simulink model "gimbal_test_2017_11_24"  (R2017a)
settings: Solver=ode14x  StartTime=0.0  StopTime=20  FixedStep=0.001  RelTol=1e-3  EnableMultiTasking=on
values from neighbouring files (symbols this model uses):
  m = MAG(:,3:5)    [acc_calibration_t1.m]
  s = tf('s')    [adaptive_control.m]    (also in constraints.m = 1e-19)
undefined symbols (not defined in the file or in its folder): sigbuilder_block, X, Y, Z
libraries: sm_lib x46, nesl_utility x35, simulink x7
(part 2 of 2)

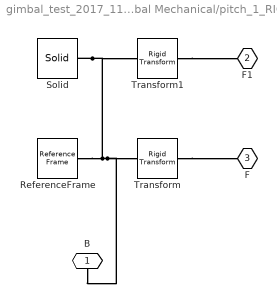
== system gimbal_test_2017_11_24/Gimbal Mechanical/pitch_1_RIGID ==
  ReferenceFrame : sm_lib/Frames and Transforms/Reference Frame
  Solid : sm_lib/Body Elements/Solid  InertiaType=Custom  Mass=0.14119942872953756  MassUnits=kg  CenterOfMass=[-40.309869373451356 137.87074734557396 -65.780666800490948]  CenterOfMassUnits=mm  MomentsOfInertia=[409.04449997922234 176.99414095993797 350.83879275246994]  MomentsOfInertiaUnits=kg*mm^2  ProductsOfInertia=[-106.85964081398967 1.9282234630967596 4.2232275028540895]  ProductsOfInertiaUnits=kg*mm^2  DensityBased=on  Density=1000  DensityUnits=kg/(m^3)  DoExposeReferenceFrame=on  SerializedFrames=<Frames/>  GraphicType=FromGeometry  MarkerShape=Sphere  MarkerSize=10  GraphicVisPropType=SimpleVisualProperties  GraphicDiffuseColor=[0.89803921568627454 0.91764705882352937 0.92941176470588238]  GraphicSpecularColor=[0.5 0.5 0.5 1.0]  GraphicAmbientColor=[0.15 0.15 0.15 1.0]  GraphicEmissiveColor=[0.0 0.0 0.0 1.0]  GraphicShininess=75  GraphicOpacity=1  GeometryShape=FromFile  RectangleSize=[1 1]  RectangleSizeUnits=m  BrickDimensions=[1 1 1]  BrickDimensionUnits=m  CylinderRadius=1  CylinderRadiusUnits=m  CylinderLength=1  CylinderLengthUnits=m  SphereRadius=1  SphereRadiusUnits=m  EllipsoidRadii=[1 1 1]  EllipsoidRadiiUnits=m  ExtrusionCrossSection=[1 1; -1 1; -1 -1; 1 -1]  ExtrusionCrossSectionUnits=m  ExtrusionLength=1  ExtrusionLengthUnits=m  PolygonNumSides=3  PolygonOuterRadius=1  PolygonOuterRadiusUnits=m  ExtGeomFileType=STEP  ExtGeomFileName=pitch_默认_sldprt.STEP  ExtGeomFileUnits=m  RevolutionCrossSection=[1 1; 1 -1; 2 -1; 2 1]  RevolutionCrossSectionUnits=m  RevolutionExtent=Full  RevolutionAngle=180  RevolutionAngleUnits=deg
  Transform : sm_lib/Frames and Transforms/Rigid Transform  TranslationMethod=Cartesian  TranslationStandardOffset=0  TranslationLengthUnit=mm  TranslationStandardAxis=+Z  TranslationCartesianOffset=[-70.90915967289996 155.67572530099997 -91.396390597699934]  TranslationROffset=0  TranslationROffsetUnits=m  TranslationZOffset=0  TranslationZOffsetUnits=m  TranslationThetaOffset=0  TranslationThetaOffsetUnits=deg  RotationMethod=ArbitraryAxis  RotationAngleUnits=rad  RotationStandardAxis=+Z  RotationAngle=0  RotationArbitraryAxis=[0 0 0]  FollAlignAxisA=+X  BaseAlignAxisA=+Y  FollAlignAxisB=+Y  BaseAlignAxisB=+Z  RotationSequenceAxes=FollowerAxes  RotationSequence=XYX  RotationSequenceAngles=[0 0 0]  RotationSequenceAnglesUnits=deg  RotationMatrix=[1 0 0; 0 1 0; 0 0 1]
  Transform1 : sm_lib/Frames and Transforms/Rigid Transform  TranslationMethod=Cartesian  TranslationStandardOffset=0  TranslationLengthUnit=mm  TranslationStandardAxis=+Z  TranslationCartesianOffset=[-38.909159672900159 1166.6150256647427 -32.030390597696254]  TranslationROffset=0  TranslationROffsetUnits=m  TranslationZOffset=0  TranslationZOffsetUnits=m  TranslationThetaOffset=0  TranslationThetaOffsetUnits=deg  RotationMethod=ArbitraryAxis  RotationAngleUnits=rad  RotationStandardAxis=+Z  RotationAngle=2.0943951023931957  RotationArbitraryAxis=[0.57735026918962595 -0.57735026918962595 0.5773502691896254]  FollAlignAxisA=+X  BaseAlignAxisA=+Y  FollAlignAxisB=+Y  BaseAlignAxisB=+Z  RotationSequenceAxes=FollowerAxes  RotationSequence=XYX  RotationSequenceAngles=[0 0 0]  RotationSequenceAnglesUnits=deg  RotationMatrix=[1 0 0; 0 1 0; 0 0 1]
  B : PMIOPort  Port=1  Side=Left
  F1 : PMIOPort  Port=2  Side=Left
  F : PMIOPort  Port=3  Side=Left
  connections:
  Solid/RConn1 -- B/RConn1 -- Transform/LConn1 -- Transform1/LConn1 -- ReferenceFrame/RConn1
  Transform/RConn1 -- F/RConn1
  Transform1/RConn1 -- F1/RConn1

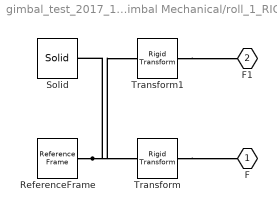
== system gimbal_test_2017_11_24/Gimbal Mechanical/roll_1_RIGID ==
  ReferenceFrame : sm_lib/Frames and Transforms/Reference Frame
  Solid : sm_lib/Body Elements/Solid  InertiaType=Custom  Mass=0.31793228993235328  MassUnits=kg  CenterOfMass=[-40.197559372662035 151.39080125157062 -75.482343271011416]  CenterOfMassUnits=mm  MomentsOfInertia=[1698.578771208184 766.33943967936329 1161.8382457192142]  MomentsOfInertiaUnits=kg*mm^2  ProductsOfInertia=[-589.52899840909799 -20.442997774547614 -29.224073948839539]  ProductsOfInertiaUnits=kg*mm^2  DensityBased=on  Density=1000  DensityUnits=kg/(m^3)  DoExposeReferenceFrame=on  SerializedFrames=<Frames/>  GraphicType=FromGeometry  MarkerShape=Sphere  MarkerSize=10  GraphicVisPropType=SimpleVisualProperties  GraphicDiffuseColor=[0.89803921568627454 0.91764705882352937 0.92941176470588238]  GraphicSpecularColor=[0.5 0.5 0.5 1.0]  GraphicAmbientColor=[0.15 0.15 0.15 1.0]  GraphicEmissiveColor=[0.0 0.0 0.0 1.0]  GraphicShininess=75  GraphicOpacity=1  GeometryShape=FromFile  RectangleSize=[1 1]  RectangleSizeUnits=m  BrickDimensions=[1 1 1]  BrickDimensionUnits=m  CylinderRadius=1  CylinderRadiusUnits=m  CylinderLength=1  CylinderLengthUnits=m  SphereRadius=1  SphereRadiusUnits=m  EllipsoidRadii=[1 1 1]  EllipsoidRadiiUnits=m  ExtrusionCrossSection=[1 1; -1 1; -1 -1; 1 -1]  ExtrusionCrossSectionUnits=m  ExtrusionLength=1  ExtrusionLengthUnits=m  PolygonNumSides=3  PolygonOuterRadius=1  PolygonOuterRadiusUnits=m  ExtGeomFileType=STEP  ExtGeomFileName=roll_默认_sldprt.STEP  ExtGeomFileUnits=m  RevolutionCrossSection=[1 1; 1 -1; 2 -1; 2 1]  RevolutionCrossSectionUnits=m  RevolutionExtent=Full  RevolutionAngle=180  RevolutionAngleUnits=deg
  Transform : sm_lib/Frames and Transforms/Rigid Transform  TranslationMethod=Cartesian  TranslationStandardOffset=0  TranslationLengthUnit=mm  TranslationStandardAxis=+Z  TranslationCartesianOffset=[-38.909159672899136 47.175725301000313 513.35498149905948]  TranslationROffset=0  TranslationROffsetUnits=m  TranslationZOffset=0  TranslationZOffsetUnits=m  TranslationThetaOffset=0  TranslationThetaOffsetUnits=deg  RotationMethod=ArbitraryAxis  RotationAngleUnits=rad  RotationStandardAxis=+Z  RotationAngle=3.1415926535897931  RotationArbitraryAxis=[-1 1.5338031114433573e-32 -2.7175667253946204e-16]  FollAlignAxisA=+X  BaseAlignAxisA=+Y  FollAlignAxisB=+Y  BaseAlignAxisB=+Z  RotationSequenceAxes=FollowerAxes  RotationSequence=XYX  RotationSequenceAngles=[0 0 0]  RotationSequenceAnglesUnits=deg  RotationMatrix=[1 0 0; 0 1 0; 0 0 1]
  Transform1 : sm_lib/Frames and Transforms/Rigid Transform  TranslationMethod=Cartesian  TranslationStandardOffset=0  TranslationLengthUnit=mm  TranslationStandardAxis=+Z  TranslationCartesianOffset=[-38.909159672900039 1167.1810510685002 -32.030390597700006]  TranslationROffset=0  TranslationROffsetUnits=m  TranslationZOffset=0  TranslationZOffsetUnits=m  TranslationThetaOffset=0  TranslationThetaOffsetUnits=deg  RotationMethod=ArbitraryAxis  RotationAngleUnits=rad  RotationStandardAxis=+Z  RotationAngle=2.0943951023931953  RotationArbitraryAxis=[0.57735026918962584 -0.57735026918962584 0.57735026918962584]  FollAlignAxisA=+X  BaseAlignAxisA=+Y  FollAlignAxisB=+Y  BaseAlignAxisB=+Z  RotationSequenceAxes=FollowerAxes  RotationSequence=XYX  RotationSequenceAngles=[0 0 0]  RotationSequenceAnglesUnits=deg  RotationMatrix=[1 0 0; 0 1 0; 0 0 1]
  F : PMIOPort  Port=1  Side=Left
  F1 : PMIOPort  Port=2  Side=Right
  connections:
  Solid/RConn1 -- ReferenceFrame/RConn1 -- Transform/LConn1 -- Transform1/LConn1
  Transform/RConn1 -- F/RConn1
  Transform1/RConn1 -- F1/RConn1

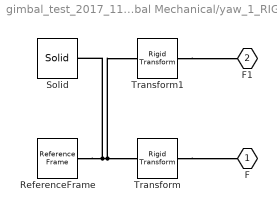
== system gimbal_test_2017_11_24/Gimbal Mechanical/yaw_1_RIGID ==
  ReferenceFrame : sm_lib/Frames and Transforms/Reference Frame
  Solid : sm_lib/Body Elements/Solid  InertiaType=Custom  Mass=0.4220224652422469  MassUnits=kg  CenterOfMass=[-39.730395407906954 147.5203430562342 -125.35459490281445]  CenterOfMassUnits=mm  MomentsOfInertia=[6109.2729904538583 920.66918616811347 5510.6384164735264]  MomentsOfInertiaUnits=kg*mm^2  ProductsOfInertia=[-1282.9600428246124 21.67357327564007 52.078346871971853]  ProductsOfInertiaUnits=kg*mm^2  DensityBased=on  Density=1000  DensityUnits=kg/(m^3)  DoExposeReferenceFrame=on  SerializedFrames=<Frames/>  GraphicType=FromGeometry  MarkerShape=Sphere  MarkerSize=10  GraphicVisPropType=SimpleVisualProperties  GraphicDiffuseColor=[0.89803921568627454 0.91764705882352937 0.92941176470588238]  GraphicSpecularColor=[0.5 0.5 0.5 1.0]  GraphicAmbientColor=[0.15 0.15 0.15 1.0]  GraphicEmissiveColor=[0.0 0.0 0.0 1.0]  GraphicShininess=75  GraphicOpacity=1  GeometryShape=FromFile  RectangleSize=[1 1]  RectangleSizeUnits=m  BrickDimensions=[1 1 1]  BrickDimensionUnits=m  CylinderRadius=1  CylinderRadiusUnits=m  CylinderLength=1  CylinderLengthUnits=m  SphereRadius=1  SphereRadiusUnits=m  EllipsoidRadii=[1 1 1]  EllipsoidRadiiUnits=m  ExtrusionCrossSection=[1 1; -1 1; -1 -1; 1 -1]  ExtrusionCrossSectionUnits=m  ExtrusionLength=1  ExtrusionLengthUnits=m  PolygonNumSides=3  PolygonOuterRadius=1  PolygonOuterRadiusUnits=m  ExtGeomFileType=STEP  ExtGeomFileName=yaw_默认_sldprt.STEP  ExtGeomFileUnits=m  RevolutionCrossSection=[1 1; 1 -1; 2 -1; 2 1]  RevolutionCrossSectionUnits=m  RevolutionExtent=Full  RevolutionAngle=180  RevolutionAngleUnits=deg
  Transform : sm_lib/Frames and Transforms/Rigid Transform  TranslationMethod=Cartesian  TranslationStandardOffset=0  TranslationLengthUnit=mm  TranslationStandardAxis=+Z  TranslationCartesianOffset=[-38.909159672899804 334.03951901900109 -32.030390597700091]  TranslationROffset=0  TranslationROffsetUnits=m  TranslationZOffset=0  TranslationZOffsetUnits=m  TranslationThetaOffset=0  TranslationThetaOffsetUnits=deg  RotationMethod=ArbitraryAxis  RotationAngleUnits=rad  RotationStandardAxis=+Z  RotationAngle=2.0943951023931962  RotationArbitraryAxis=[0.57735026918962595 -0.57735026918962562 0.57735026918962573]  FollAlignAxisA=+X  BaseAlignAxisA=+Y  FollAlignAxisB=+Y  BaseAlignAxisB=+Z  RotationSequenceAxes=FollowerAxes  RotationSequence=XYX  RotationSequenceAngles=[0 0 0]  RotationSequenceAnglesUnits=deg  RotationMatrix=[1 0 0; 0 1 0; 0 0 1]
  Transform1 : sm_lib/Frames and Transforms/Rigid Transform  TranslationMethod=Cartesian  TranslationStandardOffset=0  TranslationLengthUnit=mm  TranslationStandardAxis=+Z  TranslationCartesianOffset=[-38.909159672900067 32.039519019000039 520.28895609530014]  TranslationROffset=0  TranslationROffsetUnits=m  TranslationZOffset=0  TranslationZOffsetUnits=m  TranslationThetaOffset=0  TranslationThetaOffsetUnits=deg  RotationMethod=ArbitraryAxis  RotationAngleUnits=rad  RotationStandardAxis=+Z  RotationAngle=3.1415926535897931  RotationArbitraryAxis=[1 0 5.377642775528102e-17]  FollAlignAxisA=+X  BaseAlignAxisA=+Y  FollAlignAxisB=+Y  BaseAlignAxisB=+Z  RotationSequenceAxes=FollowerAxes  RotationSequence=XYX  RotationSequenceAngles=[0 0 0]  RotationSequenceAnglesUnits=deg  RotationMatrix=[1 0 0; 0 1 0; 0 0 1]
  F : PMIOPort  Port=1  Side=Left
  F1 : PMIOPort  Port=2  Side=Right
  connections:
  Solid/RConn1 -- ReferenceFrame/RConn1 -- Transform/LConn1 -- Transform1/LConn1
  Transform/RConn1 -- F/RConn1
  Transform1/RConn1 -- F1/RConn1

== system gimbal_test_2017_11_24/Test Bed/groud_1_RIGID ==
  ReferenceFrame : sm_lib/Frames and Transforms/Reference Frame
  Solid : sm_lib/Body Elements/Solid  InertiaType=Custom  Mass=0.744656095436107  MassUnits=kg  CenterOfMass=[0 14.834199182049298 0]  CenterOfMassUnits=mm  MomentsOfInertia=[248.52962199765179 383.88524366097863 245.75166872905808]  MomentsOfInertiaUnits=kg*mm^2  ProductsOfInertia=[0 0 0]  ProductsOfInertiaUnits=kg*mm^2  DensityBased=on  Density=1000  DensityUnits=kg/(m^3)  DoExposeReferenceFrame=on  SerializedFrames=<Frames/>  GraphicType=FromGeometry  MarkerShape=Sphere  MarkerSize=10  GraphicVisPropType=SimpleVisualProperties  GraphicDiffuseColor=[0.89411764705882346 0.9137254901960784 0.92941176470588238]  GraphicSpecularColor=[0.5 0.5 0.5 1.0]  GraphicAmbientColor=[0.15 0.15 0.15 1.0]  GraphicEmissiveColor=[0.0 0.0 0.0 1.0]  GraphicShininess=75  GraphicOpacity=1  GeometryShape=FromFile  RectangleSize=[1 1]  RectangleSizeUnits=m  BrickDimensions=[1 1 1]  BrickDimensionUnits=m  CylinderRadius=1  CylinderRadiusUnits=m  CylinderLength=1  CylinderLengthUnits=m  SphereRadius=1  SphereRadiusUnits=m  EllipsoidRadii=[1 1 1]  EllipsoidRadiiUnits=m  ExtrusionCrossSection=[1 1; -1 1; -1 -1; 1 -1]  ExtrusionCrossSectionUnits=m  ExtrusionLength=1  ExtrusionLengthUnits=m  PolygonNumSides=3  PolygonOuterRadius=1  PolygonOuterRadiusUnits=m  ExtGeomFileType=STEP  ExtGeomFileName=groud_默认_sldprt.STEP  ExtGeomFileUnits=m  RevolutionCrossSection=[1 1; 1 -1; 2 -1; 2 1]  RevolutionCrossSectionUnits=m  RevolutionExtent=Full  RevolutionAngle=180  RevolutionAngleUnits=deg
  Transform : sm_lib/Frames and Transforms/Rigid Transform  TranslationMethod=Cartesian  TranslationStandardOffset=0  TranslationLengthUnit=mm  TranslationStandardAxis=+Z  TranslationCartesianOffset=[0 30 0]  TranslationROffset=0  TranslationROffsetUnits=m  TranslationZOffset=0  TranslationZOffsetUnits=m  TranslationThetaOffset=0  TranslationThetaOffsetUnits=deg  RotationMethod=ArbitraryAxis  RotationAngleUnits=rad  RotationStandardAxis=+Z  RotationAngle=2.0943951023931953  RotationArbitraryAxis=[0.57735026918962584 -0.57735026918962584 0.57735026918962584]  FollAlignAxisA=+X  BaseAlignAxisA=+Y  FollAlignAxisB=+Y  BaseAlignAxisB=+Z  RotationSequenceAxes=FollowerAxes  RotationSequence=XYX  RotationSequenceAngles=[0 0 0]  RotationSequenceAnglesUnits=deg  RotationMatrix=[1 0 0; 0 1 0; 0 0 1]
  F1 : PMIOPort  Port=1  Side=Left
  F : PMIOPort  Port=2  Side=Right
  connections:
  Solid/RConn1 -- ReferenceFrame/RConn1 -- Transform/LConn1 -- F1/RConn1
  Transform/RConn1 -- F/RConn1

== system gimbal_test_2017_11_24/Test Bed/test_pitch_1_RIGID ==
  ReferenceFrame : sm_lib/Frames and Transforms/Reference Frame
  Solid : sm_lib/Body Elements/Solid  InertiaType=Custom  Mass=3.2542558482698221  MassUnits=kg  CenterOfMass=[0 15.000000000000004 0.00013445046945364221]  CenterOfMassUnits=mm  MomentsOfInertia=[197323.97689125084 354318.98035563418 157585.85549691919]  MomentsOfInertiaUnits=kg*mm^2  ProductsOfInertia=[0 0 0.0039657370023979469]  ProductsOfInertiaUnits=kg*mm^2  DensityBased=on  Density=1000  DensityUnits=kg/(m^3)  DoExposeReferenceFrame=on  SerializedFrames=<Frames/>  GraphicType=FromGeometry  MarkerShape=Sphere  MarkerSize=10  GraphicVisPropType=SimpleVisualProperties  GraphicDiffuseColor=[1 1 1]  GraphicSpecularColor=[0.5 0.5 0.5 1.0]  GraphicAmbientColor=[0.15 0.15 0.15 1.0]  GraphicEmissiveColor=[0.0 0.0 0.0 1.0]  GraphicShininess=75  GraphicOpacity=1  GeometryShape=FromFile  RectangleSize=[1 1]  RectangleSizeUnits=m  BrickDimensions=[1 1 1]  BrickDimensionUnits=m  CylinderRadius=1  CylinderRadiusUnits=m  CylinderLength=1  CylinderLengthUnits=m  SphereRadius=1  SphereRadiusUnits=m  EllipsoidRadii=[1 1 1]  EllipsoidRadiiUnits=m  ExtrusionCrossSection=[1 1; -1 1; -1 -1; 1 -1]  ExtrusionCrossSectionUnits=m  ExtrusionLength=1  ExtrusionLengthUnits=m  PolygonNumSides=3  PolygonOuterRadius=1  PolygonOuterRadiusUnits=m  ExtGeomFileType=STEP  ExtGeomFileName=test_pitch_默认_sldprt.STEP  ExtGeomFileUnits=m  RevolutionCrossSection=[1 1; 1 -1; 2 -1; 2 1]  RevolutionCrossSectionUnits=m  RevolutionExtent=Full  RevolutionAngle=180  RevolutionAngleUnits=deg
  Transform : sm_lib/Frames and Transforms/Rigid Transform  TranslationMethod=Cartesian  TranslationStandardOffset=0  TranslationLengthUnit=mm  TranslationStandardAxis=+Z  TranslationCartesianOffset=[0 15.000000000000568 -587]  TranslationROffset=0  TranslationROffsetUnits=m  TranslationZOffset=0  TranslationZOffsetUnits=m  TranslationThetaOffset=0  TranslationThetaOffsetUnits=deg  RotationMethod=ArbitraryAxis  RotationAngleUnits=rad  RotationStandardAxis=+Z  RotationAngle=8.3312973296909746e-16  RotationArbitraryAxis=[0.86265645032380789 -0.50579032089861853 -1.8175695005807099e-16]  FollAlignAxisA=+X  BaseAlignAxisA=+Y  FollAlignAxisB=+Y  BaseAlignAxisB=+Z  RotationSequenceAxes=FollowerAxes  RotationSequence=XYX  RotationSequenceAngles=[0 0 0]  RotationSequenceAnglesUnits=deg  RotationMatrix=[1 0 0; 0 1 0; 0 0 1]
  Transform1 : sm_lib/Frames and Transforms/Rigid Transform  TranslationMethod=Cartesian  TranslationStandardOffset=0  TranslationLengthUnit=mm  TranslationStandardAxis=+Z  TranslationCartesianOffset=[0 30 0]  TranslationROffset=0  TranslationROffsetUnits=m  TranslationZOffset=0  TranslationZOffsetUnits=m  TranslationThetaOffset=0  TranslationThetaOffsetUnits=deg  RotationMethod=ArbitraryAxis  RotationAngleUnits=rad  RotationStandardAxis=+Z  RotationAngle=2.0943951023931953  RotationArbitraryAxis=[0.57735026918962584 -0.57735026918962584 0.57735026918962584]  FollAlignAxisA=+X  BaseAlignAxisA=+Y  FollAlignAxisB=+Y  BaseAlignAxisB=+Z  RotationSequenceAxes=FollowerAxes  RotationSequence=XYX  RotationSequenceAngles=[0 0 0]  RotationSequenceAnglesUnits=deg  RotationMatrix=[1 0 0; 0 1 0; 0 0 1]
  F : PMIOPort  Port=1  Side=Left
  F1 : PMIOPort  Port=2  Side=Right
  connections:
  Solid/RConn1 -- ReferenceFrame/RConn1 -- Transform/LConn1 -- Transform1/LConn1
  Transform/RConn1 -- F/RConn1
  Transform1/RConn1 -- F1/RConn1

== system gimbal_test_2017_11_24/Test Bed/test_roll_1_RIGID ==
  ReferenceFrame : sm_lib/Frames and Transforms/Reference Frame
  Solid : sm_lib/Body Elements/Solid  InertiaType=Custom  Mass=0.20450614916336574  MassUnits=kg  CenterOfMass=[-1.0328761560106987e-05 10.226639389930648 -309.12731029151979]  CenterOfMassUnits=mm  MomentsOfInertia=[71.504553359544801 477.13713336271184 448.94842380562415]  MomentsOfInertiaUnits=kg*mm^2  ProductsOfInertia=[-0.44644966825853433 2.6790546083628789e-05 -3.8747955667632615e-05]  ProductsOfInertiaUnits=kg*mm^2  DensityBased=on  Density=1000  DensityUnits=kg/(m^3)  DoExposeReferenceFrame=on  SerializedFrames=<Frames/>  GraphicType=FromGeometry  MarkerShape=Sphere  MarkerSize=10  GraphicVisPropType=SimpleVisualProperties  GraphicDiffuseColor=[1 1 1]  GraphicSpecularColor=[0.5 0.5 0.5 1.0]  GraphicAmbientColor=[0.15 0.15 0.15 1.0]  GraphicEmissiveColor=[0.0 0.0 0.0 1.0]  GraphicShininess=75  GraphicOpacity=1  GeometryShape=FromFile  RectangleSize=[1 1]  RectangleSizeUnits=m  BrickDimensions=[1 1 1]  BrickDimensionUnits=m  CylinderRadius=1  CylinderRadiusUnits=m  CylinderLength=1  CylinderLengthUnits=m  SphereRadius=1  SphereRadiusUnits=m  EllipsoidRadii=[1 1 1]  EllipsoidRadiiUnits=m  ExtrusionCrossSection=[1 1; -1 1; -1 -1; 1 -1]  ExtrusionCrossSectionUnits=m  ExtrusionLength=1  ExtrusionLengthUnits=m  PolygonNumSides=3  PolygonOuterRadius=1  PolygonOuterRadiusUnits=m  ExtGeomFileType=STEP  ExtGeomFileName=test_roll_默认_sldprt.STEP  ExtGeomFileUnits=m  RevolutionCrossSection=[1 1; 1 -1; 2 -1; 2 1]  RevolutionCrossSectionUnits=m  RevolutionExtent=Full  RevolutionAngle=180  RevolutionAngleUnits=deg
  Transform : sm_lib/Frames and Transforms/Rigid Transform  TranslationMethod=Cartesian  TranslationStandardOffset=0  TranslationLengthUnit=mm  TranslationStandardAxis=+Z  TranslationCartesianOffset=[8.9090429904744592e-15 1.0221477966047367e-13 -1.1911909021789691e-13]  TranslationROffset=0  TranslationROffsetUnits=m  TranslationZOffset=0  TranslationZOffsetUnits=m  TranslationThetaOffset=0  TranslationThetaOffsetUnits=deg  RotationMethod=ArbitraryAxis  RotationAngleUnits=rad  RotationStandardAxis=+Z  RotationAngle=2.0943951023931953  RotationArbitraryAxis=[0.57735026918962584 -0.57735026918962629 0.57735026918962529]  FollAlignAxisA=+X  BaseAlignAxisA=+Y  FollAlignAxisB=+Y  BaseAlignAxisB=+Z  RotationSequenceAxes=FollowerAxes  RotationSequence=XYX  RotationSequenceAngles=[0 0 0]  RotationSequenceAnglesUnits=deg  RotationMatrix=[1 0 0; 0 1 0; 0 0 1]
  Transform1 : sm_lib/Frames and Transforms/Rigid Transform  TranslationMethod=Cartesian  TranslationStandardOffset=0  TranslationLengthUnit=mm  TranslationStandardAxis=+Z  TranslationCartesianOffset=[14.999999999999972 9.9999999999999947 -299.99999999999983]  TranslationROffset=0  TranslationROffsetUnits=m  TranslationZOffset=0  TranslationZOffsetUnits=m  TranslationThetaOffset=0  TranslationThetaOffsetUnits=deg  RotationMethod=ArbitraryAxis  RotationAngleUnits=rad  RotationStandardAxis=+Z  RotationAngle=0  RotationArbitraryAxis=[0 0 0]  FollAlignAxisA=+X  BaseAlignAxisA=+Y  FollAlignAxisB=+Y  BaseAlignAxisB=+Z  RotationSequenceAxes=FollowerAxes  RotationSequence=XYX  RotationSequenceAngles=[0 0 0]  RotationSequenceAnglesUnits=deg  RotationMatrix=[1 0 0; 0 1 0; 0 0 1]
  F1 : PMIOPort  Port=1  Side=Left
  F : PMIOPort  Port=2  Side=Left
  connections:
  Solid/RConn1 -- ReferenceFrame/RConn1 -- Transform/LConn1 -- Transform1/LConn1
  Transform/RConn1 -- F/RConn1
  Transform1/RConn1 -- F1/RConn1

== system gimbal_test_2017_11_24/Test Bed/test_yaw_1_RIGID ==
  ReferenceFrame : sm_lib/Frames and Transforms/Reference Frame
  Solid : sm_lib/Body Elements/Solid  InertiaType=Custom  Mass=1.613673260827966  MassUnits=kg  CenterOfMass=[-248.89867877972853 25.000221887150591 -0.00036630926726364301]  CenterOfMassUnits=mm  MomentsOfInertia=[104081.22099303995 121622.83981515096 18191.454171364006]  MomentsOfInertiaUnits=kg*mm^2  ProductsOfInertia=[-0.001740744498014553 0.078222601983178194 -0.083617721522158003]  ProductsOfInertiaUnits=kg*mm^2  DensityBased=on  Density=1000  DensityUnits=kg/(m^3)  DoExposeReferenceFrame=on  SerializedFrames=<Frames/>  GraphicType=FromGeometry  MarkerShape=Sphere  MarkerSize=10  GraphicVisPropType=SimpleVisualProperties  GraphicDiffuseColor=[1 1 1]  GraphicSpecularColor=[0.5 0.5 0.5 1.0]  GraphicAmbientColor=[0.15 0.15 0.15 1.0]  GraphicEmissiveColor=[0.0 0.0 0.0 1.0]  GraphicShininess=75  GraphicOpacity=1  GeometryShape=FromFile  RectangleSize=[1 1]  RectangleSizeUnits=m  BrickDimensions=[1 1 1]  BrickDimensionUnits=m  CylinderRadius=1  CylinderRadiusUnits=m  CylinderLength=1  CylinderLengthUnits=m  SphereRadius=1  SphereRadiusUnits=m  EllipsoidRadii=[1 1 1]  EllipsoidRadiiUnits=m  ExtrusionCrossSection=[1 1; -1 1; -1 -1; 1 -1]  ExtrusionCrossSectionUnits=m  ExtrusionLength=1  ExtrusionLengthUnits=m  PolygonNumSides=3  PolygonOuterRadius=1  PolygonOuterRadiusUnits=m  ExtGeomFileType=STEP  ExtGeomFileName=test_yaw_默认_sldprt.STEP  ExtGeomFileUnits=m  RevolutionCrossSection=[1 1; 1 -1; 2 -1; 2 1]  RevolutionCrossSectionUnits=m  RevolutionExtent=Full  RevolutionAngle=180  RevolutionAngleUnits=deg
  Transform : sm_lib/Frames and Transforms/Rigid Transform  TranslationMethod=Cartesian  TranslationStandardOffset=0  TranslationLengthUnit=mm  TranslationStandardAxis=+Z  TranslationCartesianOffset=[0 24.999999999999968 -587]  TranslationROffset=0  TranslationROffsetUnits=m  TranslationZOffset=0  TranslationZOffsetUnits=m  TranslationThetaOffset=0  TranslationThetaOffsetUnits=deg  RotationMethod=ArbitraryAxis  RotationAngleUnits=rad  RotationStandardAxis=+Z  RotationAngle=0  RotationArbitraryAxis=[0 0 0]  FollAlignAxisA=+X  BaseAlignAxisA=+Y  FollAlignAxisB=+Y  BaseAlignAxisB=+Z  RotationSequenceAxes=FollowerAxes  RotationSequence=XYX  RotationSequenceAngles=[0 0 0]  RotationSequenceAnglesUnits=deg  RotationMatrix=[1 0 0; 0 1 0; 0 0 1]
  Transform1 : sm_lib/Frames and Transforms/Rigid Transform  TranslationMethod=Cartesian  TranslationStandardOffset=0  TranslationLengthUnit=mm  TranslationStandardAxis=+Z  TranslationCartesianOffset=[-425.19949180560275 25.000000000000032 -5.6843418860808015e-14]  TranslationROffset=0  TranslationROffsetUnits=m  TranslationZOffset=0  TranslationZOffsetUnits=m  TranslationThetaOffset=0  TranslationThetaOffsetUnits=deg  RotationMethod=ArbitraryAxis  RotationAngleUnits=rad  RotationStandardAxis=+Z  RotationAngle=2.0943951023931953  RotationArbitraryAxis=[0.57735026918962562 0.57735026918962562 0.57735026918962595]  FollAlignAxisA=+X  BaseAlignAxisA=+Y  FollAlignAxisB=+Y  BaseAlignAxisB=+Z  RotationSequenceAxes=FollowerAxes  RotationSequence=XYX  RotationSequenceAngles=[0 0 0]  RotationSequenceAnglesUnits=deg  RotationMatrix=[1 0 0; 0 1 0; 0 0 1]
  F1 : PMIOPort  Port=1  Side=Left
  F : PMIOPort  Port=2  Side=Right
  connections:
  Solid/RConn1 -- ReferenceFrame/RConn1 -- Transform/LConn1 -- Transform1/LConn1
  Transform/RConn1 -- F/RConn1
  Transform1/RConn1 -- F1/RConn1

== matlab function gimbal_test_2017_11_24/Tracking ==
  data: u input; y output
function y = fcn(u)

y = u;

== matlab function gimbal_test_2017_11_24/quat to euler ==
  data: q input; euler output
function euler = quat2euler(q)
w = q(1);
x = -q(2);
y = -q(3);
z = -q(4);
euler = [asin(2*(y*z-w*x)); atan2(-2*(x*z+w*y), 2*w*w-1+2*z*z); atan2(-2*(x*y+w*z), 2*w*w-1+2*y*y)];

== matlab function gimbal_test_2017_11_24/Gimbal Mechanical/Pitch Enc ==
  data: angle input; y output; bias input
function y = enc(angle, bias)
%#codegen
while angle>pi
    angle = angle - 2*pi;
end
while angle<-pi
    angle = angle + 2*pi;
end
angle = angle + bias;
if angle>pi
    angle = angle - 2*pi;
end
if angle<-pi
    angle = angle + 2*pi;
end
y = angle;

== matlab function gimbal_test_2017_11_24/Gimbal Mechanical/Pitch Enc1 ==
  data: angle input; y output; bias input
function y = enc(angle, bias)
%#codegen
while angle>pi
    angle = angle - 2*pi;
end
while angle<-pi
    angle = angle + 2*pi;
end
angle = angle + bias;
if angle>pi
    angle = angle - 2*pi;
end
if angle<-pi
    angle = angle + 2*pi;
end
y = angle;

== matlab function gimbal_test_2017_11_24/Gimbal Mechanical/Pitch Enc2 ==
  data: angle input; y output; bias input
function y = enc(angle, bias)
%#codegen
while angle>pi
    angle = angle - 2*pi;
end
while angle<-pi
    angle = angle + 2*pi;
end
angle = angle + bias;
if angle>pi
    angle = angle - 2*pi;
end
if angle<-pi
    angle = angle + 2*pi;
end
y = angle;

== matlab function gimbal_test_2017_11_24/GradienDeclineZ ==
  data: acc input; q output; gyro input; mag input; beta_a input; beta_m input; q_ input
function q = gd(acc, gyro, mag, beta_a, beta_m, q_)
%a2e = [0;0;-1];
%m2e = [-1;0;0];
q = [1;0;0;0];
dt = 0.001;
q1 = q_(1);
q2 = q_(2);
q3 = q_(3);
q4 = q_(4);

na = norm(acc);
ax = acc(1)/na;
ay = acc(2)/na;
az = acc(3)/na;
wx = gyro(1);
wy = gyro(2);
wz = gyro(3);
nm = norm(mag);
mx = mag(1)/nm;
my = mag(2)/nm;
mz = mag(3)/nm;

f = zeros(6,1);
f(1) = -2*(q2*q4-q1*q3)-ax;
f(2) = -2*(q1*q2+q3*q4)-ay;
f(3) = -2*(0.5-q2^2-q3^2)-az;
f(4) = -2*(0.5-q3^2-q4^2)-mx;
f(5) = -2*(q2*q3-q1*q4)-my;
f(6) = -2*(q1*q3+q2*q4)-mz;
beta_f = [beta_a*f(1);
          beta_a*f(2);
          beta_a*f(3);
          beta_m*f(4);
          beta_m*f(5);
          beta_m*f(6);];
J = [2*q3   -2*q4    2*q1    -2*q2;
     -2*q2  -2*q1    -2*q4   -2*q3;
     0      4*q2     4*q3    0;
     0      0        4*q3    4*q4;
     2*q4   -2*q3    -2*q2   2*q1;
     -2*q3  -2*q4    -2*q1   -2*q2;];
df = J'*f;
ndf = norm(df);
df = df/ndf;
dbf = J'*beta_f;
ndbf = norm(dbf);
dbf = dbf/ndbf;


qdot = 0.5*[ -q2*wx - q3*wy - q4*wz;
              q1*wx + q3*wz - q4*wy;
              q1*wy - q2*wz + q4*wx;
              q1*wz + q2*wy - q3*wx;];  
          
% qdot = qdot-beta_a*df;
qdot = qdot-dbf;
q = q_+qdot*dt;

== matlab function gimbal_test_2017_11_24/quat to euler1 ==
  data: q input; euler output
function euler = quat2euler(q)
w = q(1);
x = -q(2);
y = -q(3);
z = -q(4);
euler = [asin(2*(y*z-w*x)); atan2(-2*(x*z+w*y), 2*w*w-1+2*z*z); atan2(-2*(x*y+w*z), 2*w*w-1+2*y*y)];

== matlab function gimbal_test_2017_11_24/GradienDeclineY ==
  data: acc input; q output; gyro input; mag input; beta_a input; beta_m input; q_ input
function q = gd(acc, gyro, mag, beta_a, beta_m, q_)
%a2e = [0;0;-1];
%m2e = [0;1;0];
q = [1;0;0;0];
dt = 0.001;
q1 = q_(1);
q2 = q_(2);
q3 = q_(3);
q4 = q_(4);

na = norm(acc);
ax = acc(1)/na;
ay = acc(2)/na;
az = acc(3)/na;
wx = gyro(1);
wy = gyro(2);
wz = gyro(3);
nm = norm(mag);
mx = mag(1)/nm;
my = mag(2)/nm;
mz = mag(3)/nm;

f = zeros(6,1);
f(1) = beta_a*(-2*(q2*q4-q1*q3)-ax);
f(2) = beta_a*(-2*(q1*q2+q3*q4)-ay);
f(3) = beta_a*(-2*(0.5-q2^2-q3^2)-az);
f(4) = beta_m*(2*(q1*q4+q2*q3)-mx);
f(5) = beta_m*(2*(0.5-q2^2-q4^2)-my);
f(6) = beta_m*(2*(q3*q4-q1*q2)-mz);
J = [2*q3   -2*q4    2*q1    -2*q2;
     -2*q2  -2*q1    -2*q4   -2*q3;
     0      4*q2     4*q3    0;
     2*q4    2*q3    2*q2    2*q1;
     0      -4*q2     0      -4*q4;
     -2*q2  -2*q1    2*q4    2*q3;];
df = J'*f;
ndf = norm(df);
df = df/ndf;
qdot = 0.5*[ -q2*wx - q3*wy - q4*wz;
              q1*wx + q3*wz - q4*wy;
              q1*wy - q2*wz + q4*wx;
              q1*wz + q2*wy - q3*wx;];  
          
% qdot = qdot-beta_a*df;
qdot = qdot-df;
q = q_+qdot*dt;

== matlab function gimbal_test_2017_11_24/quat to euler2 ==
  data: q input; euler output
function euler = quat2euler(q)
w = q(1);
x = -q(2);
y = -q(3);
z = -q(4);
euler = [asin(2*(y*z-w*x)); atan2(-2*(x*z+w*y), 2*w*w-1+2*z*z); atan2(-2*(x*y+w*z), 2*w*w-1+2*y*y)];

== matlab function gimbal_test_2017_11_24/Camera IMU/MATLAB Function2 ==
  data: w input; gyro output; RM input
function gyro = fcn(w, RM)
%#codegen
gyro = inv(RM)*w;

== matlab function gimbal_test_2017_11_24/Get Head from Z ==
  data: enc input; n_c output; qe2c input
function n_c = n2cam(enc,qe2c)
n = [-1;0;0];
q1 = qe2c(1);
q2 = qe2c(2);
q3 = qe2c(3);
q4 = qe2c(4);
x = enc(1);
y = enc(2);
z = enc(3);
Re2c = [2*(0.5-q3*q3-q4*q4) 2*(q1*q4+q2*q3) 2*(q2*q4-q1*q3);
        2*(q2*q3-q1*q4) 2*(0.5-q2*q2-q4*q4) 2*(q3*q4+q1*q2);
        2*(q1*q3+q2*q4) 2*(q3*q4-q1*q2) 2*(0.5-q2*q2-q3*q3)];
Oe = [1 0 0;
      0 1 0;
      0 0 0];
Rc2e = Re2c';
Tb2c = [cos(z)*cos(y)-sin(z)*sin(x)*sin(y) sin(z)*cos(y)+cos(z)*sin(x)*sin(y) -cos(x)*sin(y);
        -sin(z)*cos(x) cos(z)*cos(x) sin(x);
        cos(z)*sin(y)+sin(z)*sin(x)*cos(y) sin(z)*sin(y)-cos(z)*sin(x)*cos(y) cos(x)*cos(y)];

n_c = Re2c*Oe*Rc2e*Tb2c*n;

== matlab function gimbal_test_2017_11_24/Camera IMU/MATLAB Function1 ==
  data: a input; acc output; RM input
function acc = fcn(a, RM)
%#codegen
acc = inv(RM)*a;

== matlab function gimbal_test_2017_11_24/Camera IMU1/MATLAB Function1 ==
  data: a input; acc output; RM input
function acc = fcn(a, RM)
%#codegen
acc = inv(RM)*a;

== matlab function gimbal_test_2017_11_24/gradient decline/Madgwick ==
  data: g input; q output; a input; beta input; dt input; q_ input
function q = madgwick(g,a,beta,dt,q_)
q = [1;0;0;0];
wx = g(1);
wy = g(2);
wz = g(3);
norm_acc = norm(a);
ax = a(1)/norm_acc;
ay = a(2)/norm_acc;
az = a(3)/norm_acc;
q1 = q_(1,1);
q2 = q_(2,1);
q3 = q_(3,1);
q4 = q_(4,1);
% comput angle rate 0.5*q*w
qdot = 0.5*[ -q2*wx - q3*wy - q4*wz;
              q1*wx + q3*wz - q4*wy;
              q1*wy - q2*wz + q4*wx;
              q1*wz + q2*wy - q3*wx;];      
          
% 
% dfg = zeros(4,1);
% dfg(1,1) =  4*q1*q3*q3 + 4*q1*q2*q2 + 2*q3*ax -2*q2*ay;
% dfg(2,1) =  4*q2*q4*q4 + 4*q1*q1*q2 - 4*q2 + 8*q2^3 + 8*q2*q3*q3 - 2*q4*ax - 2*q1*ay + 4*q2*az;
% dfg(3,1) =  4*q1*q1*q3 + 4*q3*q4*q4 - 4*q3 + 8*q3*q2*q2 + 8*q3^3 + 2*q1*ax - 2*q4*ay + 4*q3*az;
% dfg(4,1) =  4*q2*q2*q4 + 4*q3*q3*q4 - 2*q2*ax - 2*q3*ay;
% dfg = dfg/norm(dfg);
% qdot = qdot-beta*dfg;

% raw equation
f = zeros(3,1);
f(1) = -2*(q2*q4-q1*q3)-ax;
f(2) = -2*(q1*q2+q3*q4)-ay;
f(3) = -2*(0.5-q2^2-q3^2)-az;
J = [2*q3   -2*q4    2*q1    -2*q2;
     -2*q2  -2*q1    -2*q4   -2*q3;
     0      4*q2     4*q3    0;];
df = J'*f;
ndf = norm(df);
df = df/ndf;
qdot = qdot-beta*df;


q = q_+qdot*dt;

== matlab function gimbal_test_2017_11_24/body att meansure/Quat body2earth ==
  data: quatb output; enc input
function quatb = quat_b2c(enc)
x2 = -enc(1)/2;
y2 = -enc(2)/2;
z2 = -enc(3)/2;
quat = zeros(1,4);
quat(1) = cos(z2)*cos(x2)*cos(y2) + sin(z2)*sin(x2)*sin(y2);
quat(2) = -cos(z2)*sin(x2)*cos(y2) - sin(z2)*cos(x2)*sin(y2);
quat(3) = -cos(z2)*cos(x2)*sin(y2) + sin(z2)*sin(x2)*cos(y2);
quat(4) = cos(z2)*sin(x2)*sin(y2) - sin(z2)*cos(x2)*cos(y2);
quatb = [quat(1) quat(2) quat(3) quat(4)];%quatmultiply(quat, quatc);

== matlab function gimbal_test_2017_11_24/body att meansure/quat product  ==
  data: a input; c output; b input
function c  = quat_pro(a, b)
c = zeros(1,4);
c(1) = a(1)*b(1) - a(2)*b(2) - a(3)*b(3) - a(4)*b(4);
c(2) = a(1)*b(2) + a(2)*b(1) + a(3)*b(4) - a(4)*b(3);
c(3) = a(1)*b(3) - a(2)*b(4) + a(3)*b(1) + a(4)*b(2);
c(4) = a(1)*b(4) + a(2)*b(3) - a(3)*b(2) + a(4)*b(1);

== matlab function gimbal_test_2017_11_24/Camera IMU1/MATLAB Function2 ==
  data: w input; gyro output; RM input
function gyro = fcn(w, RM)
%#codegen
gyro = inv(RM)*w;

== matlab function gimbal_test_2017_11_24/body att meansure/conj 1 ==
  data: q input; cq output
function cq = fcn(q)
cq = zeros(1,4);
cq(1) = q(1);
cq(2) = -q(2);
cq(3) = -q(3);
cq(4) = -q(4);

== matlab function gimbal_test_2017_11_24/body att meansure/conj 2 ==
  data: q input; cq output
function cq = fcn(q)
cq = zeros(1,4);
cq(1) = q(1);
cq(2) = -q(2);
cq(3) = -q(3);
cq(4) = -q(4);

== matlab function gimbal_test_2017_11_24/Get Head from prj  ==
  data: q input; m output; enc input
function m = head_prj(q, enc)
x = enc(1);
y = enc(2);
z = enc(3);
r1 = sin(z)*cos(y)+cos(z)*sin(x)*sin(y);
r2 = cos(z)*cos(x);
r3 = sin(z)*sin(y)-cos(z)*sin(x)*cos(y);
bx = q(1)*q(3) - q(2)*q(4);
by = -q(1)*q(2) - q(3)*q(4);
bz = q(2)*q(2) + q(3)*q(3) - 0.5;
bybz2 = bz*bz + by*by;
bxbz2 = bx*bx + bz*bz;
bxby2 = bx*bx + by*by;
bxby = bx*by;
bxbz = bx*bz;
bybz = by*bz;

m = [bybz2*r1 - bxby*r2 - bxbz*r3;
     -bxby*r1 + bxbz2*r2 - bybz*r3;
     -bxbz*r1 - bybz*r2 + bxby2*r3];

== matlab function gimbal_test_2017_11_24/Get Head from Z&X ==
  data: q input; m output; enc input
function m = head(q, enc)
ax = 2*(q(2)*q(4)-q(1)*q(3));
ay = 2*(q(1)*q(2)+q(3)*q(4));
az = 2*(0.5-q(2)^2-q(3)^2);
x = enc(1);
y = enc(2);
z = enc(3);
r12 = sin(z)*cos(y)+cos(z)*sin(x)*sin(y);
r22 = cos(z)*cos(x);
r32 = sin(z)*sin(y)-cos(z)*sin(x)*cos(y);
ar = ax*r12 + ay*r22 + az*r32;

m = [r12 - ax*ar;
     r22 - ay*ar;
     r32 - az*ar];

== matlab function gimbal_test_2017_11_24/GradienDeclineY1 ==
  data: acc input; q output; gyro input; mag input; beta_a input; beta_m input; q_ input
function q = gd(acc, gyro, mag, beta_a, beta_m, q_)
%a2e = [0;0;-1];
%m2e = [0;1;0];
q = [1;0;0;0];
dt = 0.001;
q1 = q_(1);
q2 = q_(2);
q3 = q_(3);
q4 = q_(4);

na = norm(acc);
ax = acc(1)/na;
ay = acc(2)/na;
az = acc(3)/na;
wx = gyro(1);
wy = gyro(2);
wz = gyro(3);
nm = norm(mag);
mx = mag(1)/nm;
my = mag(2)/nm;
mz = mag(3)/nm;

f = zeros(6,1);
f(1) = beta_a*(-2*(q2*q4-q1*q3)-ax);
f(2) = beta_a*(-2*(q1*q2+q3*q4)-ay);
f(3) = beta_a*(-2*(0.5-q2^2-q3^2)-az);
f(4) = beta_m*(2*(q1*q4+q2*q3)-mx);
f(5) = beta_m*(2*(0.5-q2^2-q4^2)-my);
f(6) = beta_m*(2*(q3*q4-q1*q2)-mz);
J = [2*q3   -2*q4    2*q1    -2*q2;
     -2*q2  -2*q1    -2*q4   -2*q3;
     0      4*q2     4*q3    0;
     2*q4    2*q3    2*q2    2*q1;
     0      -4*q2     0      -4*q4;
     -2*q2  -2*q1    2*q4    2*q3;];
df = J'*f;
ndf = norm(df);
df = df/ndf;
qdot = 0.5*[ -q2*wx - q3*wy - q4*wz;
              q1*wx + q3*wz - q4*wy;
              q1*wy - q2*wz + q4*wx;
              q1*wz + q2*wy - q3*wx;];  
          
% qdot = qdot-beta_a*df;
qdot = qdot-df;
q = q_+qdot*dt;

== matlab function gimbal_test_2017_11_24/quat to euler3 ==
  data: q input; euler output
function euler = quat2euler(q)
w = q(1);
x = -q(2);
y = -q(3);
z = -q(4);
euler = [asin(2*(y*z-w*x)); atan2(-2*(x*z+w*y), 2*w*w-1+2*z*z); atan2(-2*(x*y+w*z), 2*w*w-1+2*y*y)];

== matlab function gimbal_test_2017_11_24/MATLAB Function ==
  data: angle_v input; mot output; enc input
function mot = euler2mot(angle_v, enc)
x = enc(1);
y = enc(2);
ix = angle_v(1);
iy = angle_v(2);
iz = angle_v(3);

mot = [cos(y)*ix + sin(y)*iz;
       iy;%sin(y)*ix + iy + cos(y)*iz;
       -sin(y)*ix/cos(x) + cos(y)*iz/cos(x);];
